simulink model "psiupdate_new"  (R2018b)
settings: Solver=VariableStepAuto  StartTime=0.0  StopTime=10.0  RelTol=1e-3
undefined symbols (not defined in the file or in its folder): g, psi, s, Torque
settings Model: Creator=mishray  LastModifiedBy=mishray

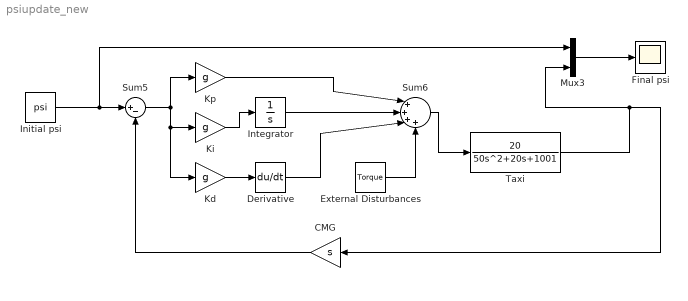
== system psiupdate_new ==
  CMG : Gain  Gain=s
  Derivative : Derivative
  External Disturbances : Constant  Value=Torque
  Final psi : Scope
  Initial psi : Constant  Value=psi
  Integrator : Integrator
  Kd : Gain  Gain=g
  Ki : Gain  Gain=g
  Kp : Gain  Gain=g
  Mux3 : Mux  Inputs=2
  Sum5 : Sum  Inputs=|+-
  Sum6 : Sum  Inputs=|++++
  Taxi : TransferFcn  Numerator=[20]  Denominator=[50 20 1001]
  wires:
  Sum5/1 -> Kd/1, Ki/1, Kp/1
  Kd/1 -> Derivative/1
  Ki/1 -> Integrator/1
  Taxi/1 -> Mux3/2, CMG/1
  CMG/1 -> Sum5/2
  Mux3/1 -> Final psi/1
  Kp/1 -> Sum6/1
  Initial psi/1 -> Mux3/1, Sum5/1
  Integrator/1 -> Sum6/2
  Derivative/1 -> Sum6/3
  External Disturbances/1 -> Sum6/4
  Sum6/1 -> Taxi/1
